simulink model "7_SCR"  (R2014a)
settings: Solver=ode23tb  StartTime=0.0  StopTime=0.08  RelTol=1e-6
libraries: powerlib x11
settings Model: Creator=CHANDRA BABU  LastModifiedBy=Divya M
settings SolverCC: ZeroCrossControl=DisableAll
settings DataIOCC: SignalLoggingSaveFormat=ModelDataLogs
settings OptimizationCC: ExpressionDepthLimit=2147483647
settings DebuggingCC: UnderspecifiedInitializationDetection=Classic  FcnCallInpInsideContextMsg=UseLocalSettings  StateNameClashWarn=warning
settings GRTTargetCC: CombineOutputUpdateFcns=off  GRTInterface=on

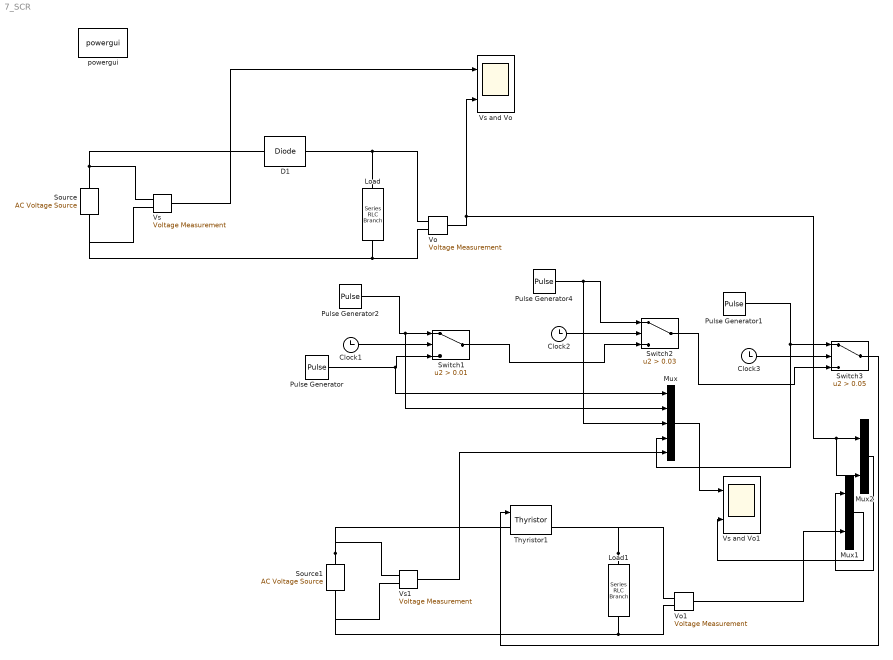
== system 7_SCR ==
  " Source" : powerlib/Electrical Sources/AC Voltage Source  Amplitude=5  Phase=0  Frequency=50  SampleTime=0  Measurements=None
  " Source1" : powerlib/Electrical Sources/AC Voltage Source  Amplitude=5  Phase=0  Frequency=50  SampleTime=0  Measurements=None
  Clock1 : Clock
  Clock2 : Clock
  Clock3 : Clock
  D1 : powerlib/Power Electronics/Diode  Ron=0.001  Lon=0  Vf=0  IC=0  UseSnubber=off  Rs=500  Cs=250e-9  Measurements=off
  Load : powerlib/Elements/Series RLC Branch  LConnTagsString=__new0  RConnTagsString=__new0  BranchType=R  Resistance=2.5  Inductance=1e-3  SetiL0=off  InitialCurrent=0  Capacitance=1e-6  Setx0=off  InitialVoltage=0  Measurements=None
  Load1 : powerlib/Elements/Series RLC Branch  LConnTagsString=__new0  RConnTagsString=__new0  BranchType=R  Resistance=2.5  Inductance=1e-3  SetiL0=off  InitialCurrent=0  Capacitance=1e-6  Setx0=off  InitialVoltage=0  Measurements=None
  Mux : Mux  Inputs=5
  Mux1 : Mux  Inputs=2
  Mux2 : Mux  Inputs=2
  Pulse Generator : DiscretePulseGenerator  PulseType=Time based  Period=0.02  PulseWidth=5
  Pulse Generator1 : DiscretePulseGenerator  PulseType=Time based  Period=0.02  PulseWidth=5  PhaseDelay=0.0075
  Pulse Generator2 : DiscretePulseGenerator  PulseType=Time based  Period=0.02  PulseWidth=5  PhaseDelay=0.0025
  Pulse Generator4 : DiscretePulseGenerator  PulseType=Time based  Period=0.02  PulseWidth=5  PhaseDelay=0.005
  Switch1 : Switch  Criteria=u2 > Threshold  Threshold=0.01
  Switch2 : Switch  Criteria=u2 > Threshold  Threshold=0.03
  Switch3 : Switch  Criteria=u2 > Threshold  Threshold=0.05
  Thyristor1 : powerlib/Power Electronics/Thyristor  Ron=0.001  Lon=0  Vf=0.8  IC=0  Rs=500  Cs=250e-9  Measurements=on
  Vo : powerlib/Measurements/Voltage Measurement  PhasorSimulation=off  OutputType=Complex  PSBequivalent=0
  Vo1 : powerlib/Measurements/Voltage Measurement  PhasorSimulation=off  OutputType=Complex  PSBequivalent=0
  Vs : powerlib/Measurements/Voltage Measurement  PhasorSimulation=off  OutputType=Complex  PSBequivalent=0
  Vs and Vo : Scope  NumInputPorts=2
      settings: YMin=-5~-5  YMax=5~5  SaveName=Outputvoltage
  Vs and Vo1 : Scope  NumInputPorts=2
      settings: YMin=-5~-5  YMax=5~5  SaveName=Outputvoltage1
  Vs1 : powerlib/Measurements/Voltage Measurement  PhasorSimulation=off  OutputType=Complex  PSBequivalent=0
  powergui : powerlib/powergui  Priority=1  SimulationMode=Continuous  SolverType=Tustin  SampleTime=50e-6  frequency=60  SPID=off  DisableSnubberDevices=off  DisableRonSwitches=off  DisableVfSwitches=off  SwTol=0  Interpol=off  DisplayEquations=off  Ts=0  methode=off  frequencyindice=0  Pbase=100e6  ErrMax=1e-4  Iterations=50  UnitsV=kV  UnitsW=MW  FunctionMessages=off  echomessages=off  HookPort=off  EnableUseOfTLC=off  x0status=blocks  RestoreLinks=warning  ResistiveCurrentMeasurement=off  Frange=[0:2:500]  Ylog=off  Xlog=on  ShowGrid=off  save=off  variable=ZData  structure=Outputvoltage  ZoomFFT=on  StartTime=0.0  cycles=1  DisplayStyle=1  fundamental=50  FreqAxis=on  MaxFrequency=1000  frequencyindicesteady=1  RmsSteady=1  display=off
  wires:
  Vs/1 -> Vs and Vo/1
  Clock1/1 -> Switch1/2
  Clock2/1 -> Switch2/2
  Pulse Generator/1 -> Mux/1, Switch1/3
  Switch1/1 -> Switch2/3
  Pulse Generator2/1 -> Mux/2, Switch1/1
  Pulse Generator4/1 -> Mux/3, Switch2/1
  Clock3/1 -> Switch3/2
  Switch2/1 -> Switch3/3
  Switch3/1 -> Thyristor1/1
  Pulse Generator1/1 -> Mux/4, Switch3/1
  Vo/1 -> Mux2/2, Mux2/1, Vs and Vo/2
  Vs1/1 -> Mux/5
  Mux/1 -> Vs and Vo1/1
  Vo1/1 -> Mux1/2
  Mux1/1 -> Vs and Vo1/2
  Mux2/1 -> Mux1/1
  connections:
  D1/LConn1 -- Vs/LConn1 -- " Source"/RConn1
  Vo/LConn1 -- D1/RConn1 -- Load/LConn1
  Vo/LConn2 -- Vs/LConn2 -- " Source"/LConn1 -- Load/RConn1
  " Source1"/RConn1 -- Thyristor1/LConn1 -- Vs1/LConn1
  Load1/LConn1 -- Thyristor1/RConn1 -- Vo1/LConn1
  Load1/RConn1 -- Vo1/LConn2 -- Vs1/LConn2 -- " Source1"/LConn1
